simulink model "SF002A_Rtn"  (R2013b)
settings: Solver=FixedStepDiscrete  SolverMode=SingleTasking  StartTime=0.0  StopTime=1  FixedStep=0.002  RelTol=1e-3
values from neighbouring files (symbols this model uses):
  ARCHGLBPRM_2MILLISEC_SEC_F32 = DataDict.Constant    [SF002A_Rtn_DataDict.m]
  FLTINJ_RTN_RTNCMD = DataDict.Constant    [SF002A_Rtn_DataDict.m]
  RtnHwAuthySlew = DataDict.Calibration    [SF002A_Rtn_DataDict.m]
  RtnOffsRng = DataDict.Calibration    [SF002A_Rtn_DataDict.m]
  RtnOffsSlew = DataDict.Calibration    [SF002A_Rtn_DataDict.m]
libraries: FloatToFixd x8, FixdToFloat x5, NxtrLim x4, NxtrAbslt x3, BilnrIntrpnMplX x3, LnrIntrpn x2, simulink x1, NxtrSign x1
settings Model: Creator=tz5743  LastModifiedBy=XZB1DB
settings SolverCC: AutoInsertRateTranBlk=on  InsertRTBMode=Always
settings DataIOCC: LimitDataPoints=off  SaveFormat=Structure  ReturnWorkspaceOutputs=on
settings OptimizationCC: BlockReduction=off  InlineParams=on  ZeroExternalMemoryAtStartup=off  ZeroInternalMemoryAtStartup=off  OptimizeModelRefInitCode=on  LifeSpan=1
settings DebuggingCC: SignalInfNanChecking=error  SignalRangeChecking=warning  UnderspecifiedInitializationDetection=Simplified  SolverPrmCheckMsg=error  InheritedTsInSrcMsg=error  DiscreteInheritContinuousMsg=error  SingleTaskRateTransMsg=error  TasksWithSamePriorityMsg=error  SigSpecEnsureSampleTimeMsg=error  CheckMatrixSingularityMsg=error  ParameterUnderflowMsg=error  ParameterPrecisionLossMsg=error  ParameterTunabilityLossMsg=error  FixptConstUnderflowMsg=warning  FixptConstOverflowMsg=warning  VectorMatrixConversionMsg=error  SignalLabelMismatchMsg=error  UnconnectedInputMsg=error  UnconnectedOutputMsg=error  UnconnectedLineMsg=error  SFcnCompatibilityMsg=error  UniqueDataStoreMsg=warning  BusObjectLabelMismatch=error  RootOutportRequireBusObject=error  AssertControl=DisableAll  ModelReferenceIOMsg=error  ModelReferenceVersionMismatchMessage=warning  ModelReferenceIOMismatchMessage=error  ModelReferenceCSMismatchMessage=warning  ModelReferenceDataLoggingMessage=error  StateNameClashWarn=warning  StrictBusMsg=ErrorOnBusTreatedAsVector  NonBusSignalsTreatedAsBus=error  SFUnexpectedBacktrackingDiag=error  SFInvalidInputDataAccessInChartInitDiag=error  SFNoUnconditionalDefaultTransitionDiag=error  SFTransitionOutsideNaturalParentDiag=error  SFUnconditionalTransitionShadowingDiag=error  SFUndirectedBroadcastEventsDiag=error
settings ModelReferenceCC: ModelReferenceNumInstancesAllowed=Single
settings RTWCC: SystemTargetFile=autosar.tlc  GenCodeOnly=on  TemplateMakefile=ert_default_tmf  Description=AUTOSAR  GenerateReport=on  ProcessScript=autosar_make_rtw_hook  LaunchReport=on
settings CodeAppCC: GenerateComments=off  IgnoreCustomStorageClasses=off  CustomSymbolStrType=$N$R$M  CustomSymbolStrBlkIO=$N$M  SimulinkBlockComments=off
settings STFCustomTargetCC: ParMdlRefBuildCompliant=on  CompOptLevelCompliant=on  IncludeMdlTerminateFcn=off  CombineOutputUpdateFcns=on  SuppressErrorStatus=on  ERTFirstTimeCompliant=on  ERTCustomFileBanners=on  SupportNonFinite=off  SupportComplex=off  SupportContinuousTime=off  SupportNonInlinedSFcns=off  MATLABClassNameForMDSCustomization=Simulink.SoftwareTarget.ERTCustomization  AutosarCompliant=on  GRTInterface=off  SystemTargetFile=autosar.tlc
settings ERTTargetCC: CodeReplacementLibrary=ANSI_C  ConcurrentExecutionCompliant=off  IncludeMdlTerminateFcn=off  SuppressErrorStatus=on  SupportNonFinite=off  SupportComplex=off  ModelStepFunctionPrototypeControlCompliant=off  CPPClassGenCompliant=off  AutosarCompliant=on  InlinedParameterPlacement=NonHierarchical  ERTCustomFileTemplate=example_file_process.tlc  EnableUserReplacementTypes=on

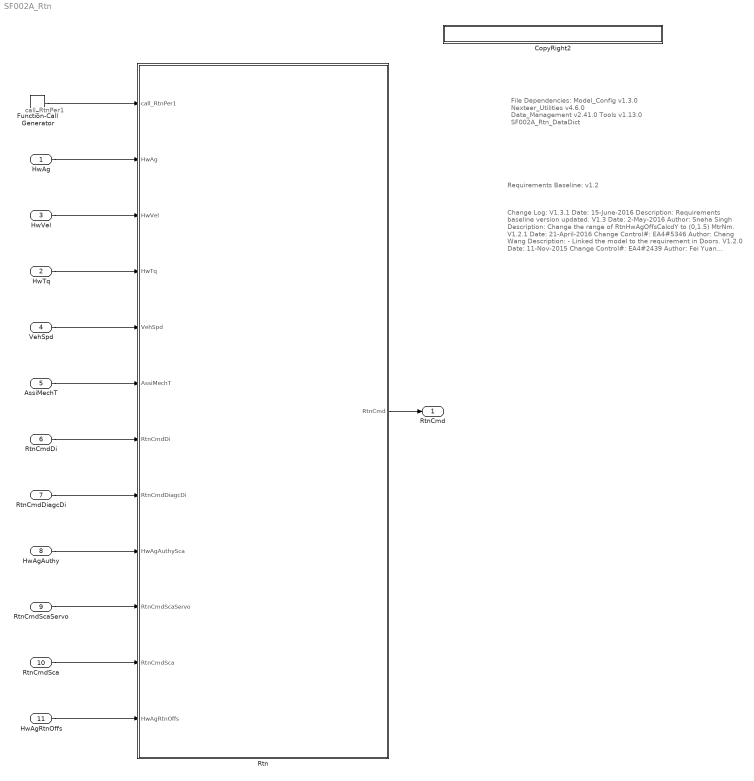
== system SF002A_Rtn ==
  note: call_RtnPer1
  note: File Dependencies:
      |
      | Model_Config v1.3.0
      | Nexteer_Utilities v4.6.0
      | Data_Management v2.41.0
      | Tools v1.13.0
      | SF002A_Rtn_DataDict
  note: Requirements Baseline: v1.2
  note: Change Log:
      |
      | V1.3.1
      | Date: 15-June-2016
      | Description:
      | Requirements baseline version updated.
      |
      | V1.3
      | Date: 2-May-2016
      | Author: Sneha Singh
      | Description:
      | Change the range of RtnHwAgOffsCalcdY to
      | (0,1.5) MtrNm.
      |
      | V1.2.1
      | Date: 21-April-2016
      | Change Control#: EA4#5346
      | Author: Chang Wang
      | Description:
      | - Linked the model to the requirement in Doors.
      |
      | V1.2.0
      | Date: 11-Nov-2015
      | Change Control#: EA4#2439
      | Author: Fei Yuan
      | Description:
      | Change the initial value of RtnCmdScaServo to 1
      |
      | V1.1.0
      | Date:29-Oct-2015
      | Change Control#: EA4#2248
      | Author : Sudeep Shankar
      | Description:
      | HwTq and HwVel changed to absolute values
      | before float to unsigned int conversion to fix
      | floating point error.
      |
      | v1.0.0
      | Date: 18-Jun-2015
      | Change Control #: EA4#759
      | DRW:  Sudeep Shankar
      | Description:
      | - Initial Release
  HwAg : Inport  RequirementInfo={'linktype_rmi_doors' '0000a524 (/E-STEER Core/SubSystem Specifications/Application Functions/SF002A Return)' '#SF002A_159' 'true' 'REQ:SF002A_159' '' } %GIDa_ca9d562d_6fa6_4620_b7e9_0be4ef6b3256
  HwTq : Inport  RequirementInfo={'linktype_rmi_doors' '0000a524 (/E-STEER Core/SubSystem Specifications/Application Functions/SF002A Return)' '#SF002A_161' 'true' 'REQ:SF002A_161' '' } %GIDa_270472cb_7f1b_499d_b316_9d3a4d63b4ae  Port=2
  HwVel : Inport  RequirementInfo={'linktype_rmi_doors' '0000a524 (/E-STEER Core/SubSystem Specifications/Application Functions/SF002A Return)' '#SF002A_160' 'true' 'REQ:SF002A_160' '' } %GIDa_baf48a56_f0cb_4bf9_a471_e23550366fc3  Port=3
  VehSpd : Inport  RequirementInfo={'linktype_rmi_doors' '0000a524 (/E-STEER Core/SubSystem Specifications/Application Functions/SF002A Return)' '#SF002A_162' 'true' 'REQ:SF002A_162' '' } %GIDa_bbc4534a_439c_4303_b734_20c92152eed5  Port=4
  AssiMechT : Inport  RequirementInfo={'linktype_rmi_doors' '0000a524 (/E-STEER Core/SubSystem Specifications/Application Functions/SF002A Return)' '#SF002A_163' 'true' 'REQ:SF002A_163' '' } %GIDa_7c5d29d7_e5a1_483a_8b5e_5f7fb39cc9db  Port=5
  RtnCmdDi : Inport  RequirementInfo={'linktype_rmi_doors' '0000a524 (/E-STEER Core/SubSystem Specifications/Application Functions/SF002A Return)' '#SF002A_164' 'true' 'REQ:SF002A_164' '' } %GIDa_de28c24d_f087_49cf_b2a4_d8c99114b430  Port=6
  RtnCmdDiagcDi : Inport  RequirementInfo={'linktype_rmi_doors' '0000a524 (/E-STEER Core/SubSystem Specifications/Application Functions/SF002A Return)' '#SF002A_165' 'true' 'REQ:SF002A_165' '' } %GIDa_ba846f76_0715_4d73_996c_66d22bdcf12b  Port=7
  HwAgAuthy : Inport  RequirementInfo={'linktype_rmi_doors' '0000a524 (/E-STEER Core/SubSystem Specifications/Application Functions/SF002A Return)' '#SF002A_166' 'true' 'REQ:SF002A_166' '' } %GIDa_5832e332_1aac_4b18_b389_bf82018842e7  Port=8
  RtnCmdScaServo : Inport  RequirementInfo={'linktype_rmi_doors' '0000a524 (/E-STEER Core/SubSystem Specifications/Application Functions/SF002A Return)' '#SF002A_167' 'true' 'REQ:SF002A_167' '' } %GIDa_ed132ec2_d50e_44ae_b5b8_67025ec0ffe6  Port=9
  RtnCmdSca : Inport  RequirementInfo={'linktype_rmi_doors' '0000a524 (/E-STEER Core/SubSystem Specifications/Application Functions/SF002A Return)' '#SF002A_168' 'true' 'REQ:SF002A_168' '' } %GIDa_5ecd380a_25d4_4e78_abc9_382ca1348921  Port=10
  HwAgRtnOffs : Inport  RequirementInfo={'linktype_rmi_doors' '0000a524 (/E-STEER Core/SubSystem Specifications/Application Functions/SF002A Return)' '#SF002A_169' 'true' 'REQ:SF002A_169' '' } %GIDa_4cf8cc8a_4d33_4739_b48e_beac64132d5a  Port=11
  CopyRight2 : Subsystem  Description=|  mask(Copyright Information){none=on}
      | Copyright info block.                                               
      |                                                                     
      | Place copyright information at the top of every subsystem in design.
      mask prompts: none "No parameters"
      mask help: Place copyright information at the top of every subsystem in design.
      mask Display:
      | NxtrConf = 'Nexteer Confidential';
      | 
      | sys = bdroot; %handle for the current model ("system")
      | first = get_param(sys,'Created');
      | if(isempty(first))
      |     first = datestr(now,'yyyy');
      | else
      |     first = first(end-3:end);  %year is last four digits
      | end
      | 
      | last = get_param(sys,'LastModifiedDate');
      | if isempty(last)
      |     last = datestr(now,'yyyy');
      | else
      |     last = last(end-3:end);
      | end
      | 
      | if strcmp(first,last)
      |     fprintf('%s -- Copyright %s Nexteer',NxtrConf,first)
      | else
      |     fprintf('%s -- %s%s- %s Nexteer',NxtrConf,char(169),first,last)
      | end
  Function-Call Generator : simulink/Ports & Subsystems/Function-Call Generator  RequirementInfo={} %GIDa_69592b82_c58d_4ec1_9fe3_c081b0261161  sample_time=0.002  numberOfIterations=1
  Rtn : Subsystem
  RtnCmd : Outport  RequirementInfo={'linktype_rmi_doors' '0000a524 (/E-STEER Core/SubSystem Specifications/Application Functions/SF002A Return)' '#SF002A_171' 'true' 'REQ:SF002A_171' '' } %GIDa_32987518_840e_4738_ba6a_c375293d3a7a
  wires:
  HwAg/1 -> Rtn/2(HwAg)
  HwVel/1 -> Rtn/3(HwVel)
  HwTq/1 -> Rtn/4(HwTq)
  VehSpd/1 -> Rtn/5(VehSpd)
  AssiMechT/1 -> Rtn/6(AssiMechT)
  RtnCmdDi/1 -> Rtn/7(RtnCmdDi)
  RtnCmdDiagcDi/1 -> Rtn/8(RtnCmdDiagcDi)
  HwAgAuthy/1 -> Rtn/9(HwAgAuthySca)
  RtnCmdScaServo/1 -> Rtn/10(RtnCmdScaServo)
  RtnCmdSca/1 -> Rtn/11(RtnCmdSca)
  HwAgRtnOffs/1 -> Rtn/12(HwAgRtnOffs)
  Rtn/1(RtnCmd) -> RtnCmd/1
  Function-Call Generator/1 -> Rtn/1(call_RtnPer1)

== system SF002A_Rtn/CopyRight2 ==

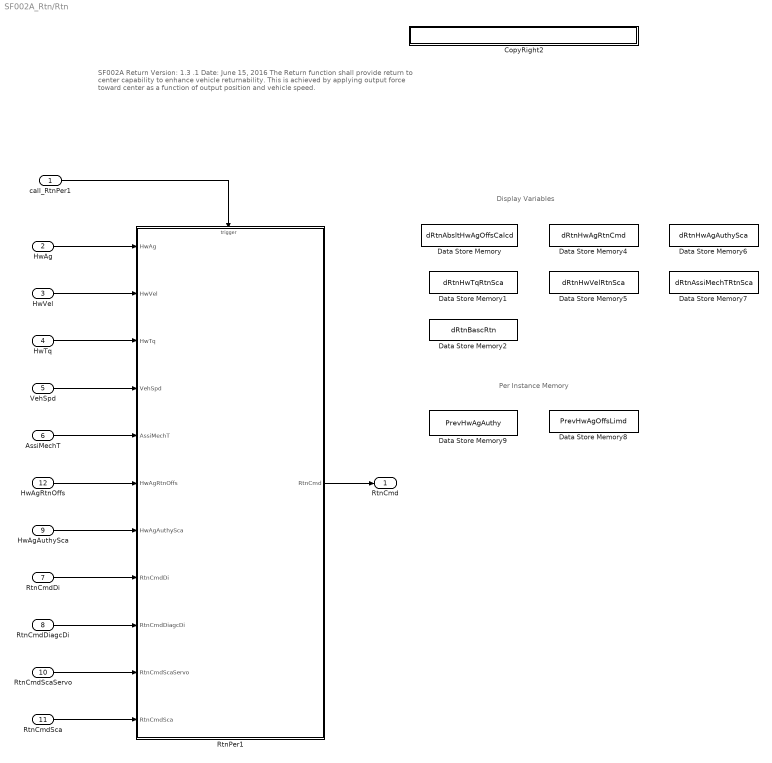
== system SF002A_Rtn/Rtn ==
  note: Per Instance Memory
  note: Display Variables
  note: SF002A Return       Version: 1.3 .1                                                    Date: June 15, 2016
      |
      | The Return function shall provide return to center capability to enhance vehicle returnability.
      | This is achieved by applying output force toward center as a function of output position and
      | vehicle speed.
  call_RtnPer1 : Inport
  HwAg : Inport  RequirementInfo={} %GIDa_81f6b954_2096_4808_9308_111896067df5  Port=2
  HwVel : Inport  RequirementInfo={} %GIDa_c3703c3f_c0e7_449a_8c9c_49994e2a0764  Port=3
  HwTq : Inport  RequirementInfo={} %GIDa_5aef1dee_ffa2_4027_a66e_3b3fd1650829  Port=4
  VehSpd : Inport  RequirementInfo={} %GIDa_5b3b3cf4_de38_4bc4_96c0_03a7b893fecb  Port=5
  AssiMechT : Inport  RequirementInfo={} %GIDa_63965e99_8cd9_4f5a_a8f1_ab380e00a545  Port=6
  RtnCmdDi : Inport  RequirementInfo={} %GIDa_5f11c497_b3cf_4940_a418_441be7e406df  Port=7
  RtnCmdDiagcDi : Inport  RequirementInfo={} %GIDa_42044fc9_5ea7_4c65_87aa_626e1dc46c63  Port=8
  HwAgAuthySca : Inport  RequirementInfo={} %GIDa_9af6312e_2c94_46c3_8264_c004198b3d25  Port=9
  RtnCmdScaServo : Inport  RequirementInfo={} %GIDa_cf95d922_a662_4add_b87b_c0abf245239e  Port=10
  RtnCmdSca : Inport  RequirementInfo={} %GIDa_d5119aae_365f_4c0e_b544_e70e493d88e1  Port=11
  HwAgRtnOffs : Inport  RequirementInfo={} %GIDa_3b2239f5_93a1_48f2_b8ad_42fbfe65ccd3  Port=12
  CopyRight2 : Subsystem  Description=|  mask(Copyright Information){none=on}
      | Copyright info block.                                               
      |                                                                     
      | Place copyright information at the top of every subsystem in design.
      mask prompts: none "No parameters"
      mask help: Place copyright information at the top of every subsystem in design.
      mask Display:
      | NxtrConf = 'Nexteer Confidential';
      | 
      | sys = bdroot; %handle for the current model ("system")
      | first = get_param(sys,'Created');
      | if(isempty(first))
      |     first = datestr(now,'yyyy');
      | else
      |     first = first(end-3:end);  %year is last four digits
      | end
      | 
      | last = get_param(sys,'LastModifiedDate');
      | if isempty(last)
      |     last = datestr(now,'yyyy');
      | else
      |     last = last(end-3:end);
      | end
      | 
      | if strcmp(first,last)
      |     fprintf('%s -- Copyright %s Nexteer',NxtrConf,first)
      | else
      |     fprintf('%s -- %s%s- %s Nexteer',NxtrConf,char(169),first,last)
      | end
  Data Store Memory : DataStoreMemory  DataStoreName=dRtnAbsltHwAgOffsCalcd  ReadBeforeWriteMsg=warning  WriteAfterWriteMsg=warning  WriteAfterReadMsg=warning  StateMustResolveToSignalObject=on
  Data Store Memory1 : DataStoreMemory  DataStoreName=dRtnHwTqRtnSca  ReadBeforeWriteMsg=warning  WriteAfterWriteMsg=warning  WriteAfterReadMsg=warning  StateMustResolveToSignalObject=on
  Data Store Memory2 : DataStoreMemory  DataStoreName=dRtnBascRtn  ReadBeforeWriteMsg=warning  WriteAfterWriteMsg=warning  WriteAfterReadMsg=warning  StateMustResolveToSignalObject=on
  Data Store Memory4 : DataStoreMemory  DataStoreName=dRtnHwAgRtnCmd  ReadBeforeWriteMsg=warning  WriteAfterWriteMsg=warning  WriteAfterReadMsg=warning  StateMustResolveToSignalObject=on
  Data Store Memory5 : DataStoreMemory  DataStoreName=dRtnHwVelRtnSca  ReadBeforeWriteMsg=warning  WriteAfterWriteMsg=warning  WriteAfterReadMsg=warning  StateMustResolveToSignalObject=on
  Data Store Memory6 : DataStoreMemory  DataStoreName=dRtnHwAgAuthySca  ReadBeforeWriteMsg=warning  WriteAfterWriteMsg=warning  WriteAfterReadMsg=warning  StateMustResolveToSignalObject=on
  Data Store Memory7 : DataStoreMemory  DataStoreName=dRtnAssiMechTRtnSca  ReadBeforeWriteMsg=warning  WriteAfterWriteMsg=warning  WriteAfterReadMsg=warning  StateMustResolveToSignalObject=on
  Data Store Memory8 : DataStoreMemory  DataStoreName=PrevHwAgOffsLimd  StateMustResolveToSignalObject=on
  Data Store Memory9 : DataStoreMemory  DataStoreName=PrevHwAgAuthy  StateMustResolveToSignalObject=on
  RtnPer1 : Subsystem  TreatAsAtomicUnit=on
  RtnCmd : Outport  RequirementInfo={} %GIDa_05e2840d_7433_4fe4_a387_0e6fe9f74771
  wires:
  AssiMechT/1 -> RtnPer1/5(AssiMechT)
  HwAgRtnOffs/1 -> RtnPer1/6(HwAgRtnOffs)
  RtnPer1/1(RtnCmd) -> RtnCmd/1
  HwAg/1 -> RtnPer1/1(HwAg)
  VehSpd/1 -> RtnPer1/4(VehSpd)
  HwTq/1 -> RtnPer1/3(HwTq)
  HwVel/1 -> RtnPer1/2(HwVel)
  call_RtnPer1/1 -> RtnPer1/Trigger
  HwAgAuthySca/1 -> RtnPer1/7(HwAgAuthySca)
  RtnCmdDi/1 -> RtnPer1/8(RtnCmdDi)
  RtnCmdDiagcDi/1 -> RtnPer1/9(RtnCmdDiagcDi)
  RtnCmdSca/1 -> RtnPer1/11(RtnCmdSca)
  RtnCmdScaServo/1 -> RtnPer1/10(RtnCmdScaServo)

== system SF002A_Rtn/Rtn/CopyRight2 ==

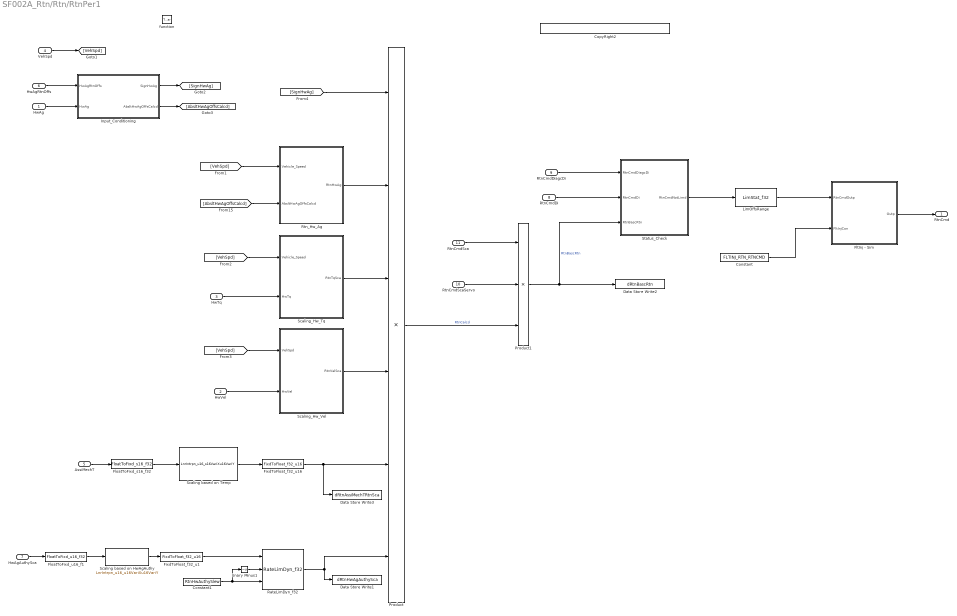
== system SF002A_Rtn/Rtn/RtnPer1 ==
  HwAg : Inport
  HwVel : Inport  Port=2
  HwTq : Inport  Port=3
  VehSpd : Inport  Port=4
  AssiMechT : Inport  Port=5
  HwAgRtnOffs : Inport  Port=6
  HwAgAuthySca : Inport  Port=7
  RtnCmdDi : Inport  Port=8
  RtnCmdDiagcDi : Inport  Port=9
  RtnCmdScaServo : Inport  Port=10
  RtnCmdSca : Inport  Port=11
  function : TriggerPort  TriggerType=function-call
  Constant : Constant  Value=FLTINJ_RTN_RTNCMD
  Constant1 : Constant  RequirementInfo={'linktype_rmi_doors' '0000a524 (/E-STEER Core/SubSystem Specifications/Application Functions/SF002A Return)' '#SF002A_206' 'true' 'REQ:SF002A_206' '' } %GIDa_f29b5096_6a10_4d8c_aa2b_ab6d9dbc01dd  Value=RtnHwAuthySlew
  CopyRight2 : Subsystem  Description=|  mask(Copyright Information){none=on}
      | Copyright info block.                                               
      |                                                                     
      | Place copyright information at the top of every subsystem in design.
      mask prompts: none "No parameters"
      mask help: Place copyright information at the top of every subsystem in design.
      mask Display:
      | NxtrConf = 'Nexteer Confidential';
      | 
      | sys = bdroot; %handle for the current model ("system")
      | first = get_param(sys,'Created');
      | if(isempty(first))
      |     first = datestr(now,'yyyy');
      | else
      |     first = first(end-3:end);  %year is last four digits
      | end
      | 
      | last = get_param(sys,'LastModifiedDate');
      | if isempty(last)
      |     last = datestr(now,'yyyy');
      | else
      |     last = last(end-3:end);
      | end
      | 
      | if strcmp(first,last)
      |     fprintf('%s -- Copyright %s Nexteer',NxtrConf,first)
      | else
      |     fprintf('%s -- %s%s- %s Nexteer',NxtrConf,char(169),first,last)
      | end
  Data Store Write1 : DataStoreWrite  DataStoreName=dRtnHwAgAuthySca
  Data Store Write2 : DataStoreWrite  DataStoreName=dRtnBascRtn
  Data Store Write3 : DataStoreWrite  DataStoreName=dRtnAssiMechTRtnSca
  FixdToFloat_f32_u1 : FixdToFloat/FixdToFloat_f32_u16  RequirementInfo={'linktype_rmi_doors' '0000a524 (/E-STEER Core/SubSystem Specifications/Application Functions/SF002A Return)' '#SF002A_205' 'true' 'REQ:SF002A_205' '' } %GIDa_b2f13837_bf2e_4759_92c8_f7ebb739a05c  Param1=7
  FixdToFloat_f32_u16 : FixdToFloat/FixdToFloat_f32_u16  RequirementInfo={'linktype_rmi_doors' '0000a524 (/E-STEER Core/SubSystem Specifications/Application Functions/SF002A Return)' '#SF002A_204' 'true' 'REQ:SF002A_204' '' } %GIDa_82025f1b_559c_4aab_bbbd_02cf94200a87  Param1=8
  FloatToFixd_s16_f32 : FloatToFixd/FloatToFixd_s16_f32  RequirementInfo={'linktype_rmi_doors' '0000a524 (/E-STEER Core/SubSystem Specifications/Application Functions/SF002A Return)' '#SF002A_204' 'true' 'REQ:SF002A_204' '' } %GIDa_56e826a7_394e_467a_81db_778c5b532e30  Param1=4
  FloatToFixd_u16_f1 : FloatToFixd/FloatToFixd_u16_f32  RequirementInfo={'linktype_rmi_doors' '0000a524 (/E-STEER Core/SubSystem Specifications/Application Functions/SF002A Return)' '#SF002A_205' 'true' 'REQ:SF002A_205' '' } %GIDa_026014ca_9083_4924_b7c0_5d559a60553d  Param1=8
  FltInj - Sim : Subsystem  TreatAsAtomicUnit=on  VariantControl=FltInj_sim  mask(Fault_Injection){}
      mask help: Fault Injection is a simulation only block for EA4 programs.
  Input_Conditioning : Subsystem  RequirementInfo={} %GIDa_067d012a_6457_4c55_9353_da0c0471b184
  LimOffsRange : NxtrLim/LimStat_f32  RequirementInfo={'linktype_rmi_doors' '0000a524 (/E-STEER Core/SubSystem Specifications/Application Functions/SF002A Return)' '#SF002A_212' 'true' 'REQ:SF002A_212' '' ; 'linktype_rmi_doors' '0000a524 (/E-STEER Core/SubSystem Specifications/Application Functions/SF002A Return)' '#SF002A_213' 'true' 'REQ:SF002A_213' '' } %GIDa_ab23da02_3b34_46cd_b196_7f8073eb848d  LoLim=SYSGLBPRM_MOTTQCMDLOLIM_MOTNWTMTR_F32  HiLim=SYSGLBPRM_MOTTQCMDHILIM_MOTNWTMTR_F32
      settings: AttributesFormatString=|
      | Low Limit: %<LoLim>
      | High Limit:%<HiLim>
  Product : Product  RequirementInfo={'linktype_rmi_doors' '0000a524 (/E-STEER Core/SubSystem Specifications/Application Functions/SF002A Return)' '#SF002A_207' 'true' 'REQ:SF002A_207' '' ; 'linktype_rmi_doors' '0000a524 (/E-STEER Core/SubSystem Specifications/Application Functions/SF002A Return)' '#SF002A_208' 'true' 'REQ:SF002A_208' '' } %GIDa_08f8f894_2fa8_4f72_bac9_f7575f211a8c  Inputs=6  RndMeth=Zero
  Product1 : Product  RequirementInfo={'linktype_rmi_doors' '0000a524 (/E-STEER Core/SubSystem Specifications/Application Functions/SF002A Return)' '#SF002A_207' 'true' 'REQ:SF002A_207' '' } %GIDa_71e52ba4_2843_42bc_8970_a10228086c20  Inputs=3  RndMeth=Zero
  RateLimDyn_f32 : NxtrLim/RateLimDyn_f32  RequirementInfo={'linktype_rmi_doors' '0000a524 (/E-STEER Core/SubSystem Specifications/Application Functions/SF002A Return)' '#SF002A_206' 'true' 'REQ:SF002A_206' '' } %GIDa_b7a544e9_f336_4c69_9d45_b0b4739fef51  StVar=PrevHwAgAuthy  Ts=ARCHGLBPRM_2MILLISEC_SEC_F32
      settings: AttributesFormatString=StVar: %<StVar>
  Rtn_Hw_Ag : Subsystem
  Scaling based on HwAgAuthy : LnrIntrpn/LnrIntrpn_u16_u16VariXu16VariY  RequirementInfo={'linktype_rmi_doors' '0000a524 (/E-STEER Core/SubSystem Specifications/Application Functions/SF002A Return)' '#SF002A_205' 'true' 'REQ:SF002A_205' '' } %GIDa_a2e059e5_fe33_4929_8913_41229897d28b  XTbl=RtnHwAuthyScaX  YTbl=RtnHwAuthyScaY
      settings: AttributesFormatString=Lnr ( u16VariX , u16VariY )
  Scaling based on Temp : LnrIntrpn/LnrIntrpn_u16_s16VariXu16VariY  RequirementInfo={'linktype_rmi_doors' '0000a524 (/E-STEER Core/SubSystem Specifications/Application Functions/SF002A Return)' '#SF002A_204' 'true' 'REQ:SF002A_204' '' } %GIDa_a7aa3a35_56d3_48d3_9473_6da7fb71fcbd  XTbl=RtnTScaX  YTbl=RtnTScaY
      settings: AttributesFormatString=Lnr ( s16VariX , u16VariY )
  Scaling_Hw_Tq : Subsystem
  Scaling_Hw_Vel : Subsystem
  Status_Check : Subsystem
  Unary Minus1 : UnaryMinus  RequirementInfo={'linktype_rmi_doors' '0000a524 (/E-STEER Core/SubSystem Specifications/Application Functions/SF002A Return)' '#SF002A_206' 'true' 'REQ:SF002A_206' '' } %GIDa_c50e97ce_443b_433d_b8c3_12b3522cf517
  RtnCmd : Outport
  wires:
  VehSpd/1 -> [VehSpd]
  HwAgRtnOffs/1 -> Input_Conditioning/1(HwAgRtnOffs)
  HwAg/1 -> Input_Conditioning/2(HwAg)
  Input_Conditioning/2(AbsltHwAgOffsCalcd) -> [AbsltHwAgOffsCalcd]
  Input_Conditioning/1(SignHwAg) -> [SignHwAg]
  [VehSpd] -> Rtn_Hw_Ag/1(Vehicle_Speed)
  [AbsltHwAgOffsCalcd] -> Rtn_Hw_Ag/2(AbsltHwAgOffsCalcd)
  [VehSpd] -> Scaling_Hw_Tq/1(Vehicle_Speed)
  HwTq/1 -> Scaling_Hw_Tq/2(HwTq)
  HwVel/1 -> Scaling_Hw_Vel/2(HwVel)
  [VehSpd] -> Scaling_Hw_Vel/1(VehSpd)
  [SignHwAg] -> Product/1
  Rtn_Hw_Ag/1(RtnHwAg) -> Product/2
  Scaling_Hw_Tq/1(RtnTqSca) -> Product/3
  Scaling_Hw_Vel/1(RtnVelSca) -> Product/4
  Scaling based on Temp/1 -> FixdToFloat_f32_u16/1
  RateLimDyn_f32/1 -> Product/6, Data Store Write1/1
  RtnCmdScaServo/1 -> Product1/2
  RtnCmdSca/1 -> Product1/1
  Product/1 -> Product1/3  "RtnCalcd"
  RtnCmdDiagcDi/1 -> Status_Check/1(RtnCmdDiagcDi)
  RtnCmdDi/1 -> Status_Check/2(RtnCmdDi)
  Product1/1 -> Data Store Write2/1, Status_Check/3(RtnBascRtn)  "RtnBascRtn"
  Status_Check/1(RtnCmdNotLimd) -> LimOffsRange/1
  AssiMechT/1 -> FloatToFixd_s16_f32/1
  FixdToFloat_f32_u16/1 -> Data Store Write3/1, Product/5
  FloatToFixd_s16_f32/1 -> Scaling based on Temp/1
  HwAgAuthySca/1 -> FloatToFixd_u16_f1/1
  FloatToFixd_u16_f1/1 -> Scaling based on HwAgAuthy/1
  Scaling based on HwAgAuthy/1 -> FixdToFloat_f32_u1/1
  FixdToFloat_f32_u1/1 -> RateLimDyn_f32/1
  Unary Minus1/1 -> RateLimDyn_f32/2
  Constant1/1 -> RateLimDyn_f32/3, Unary Minus1/1
  LimOffsRange/1 -> FltInj - Sim/1(RtnCmdOutp)
  FltInj - Sim/1(Outp) -> RtnCmd/1
  Constant/1 -> FltInj - Sim/2(FltInjCon)

== system SF002A_Rtn/Rtn/RtnPer1/CopyRight2 ==

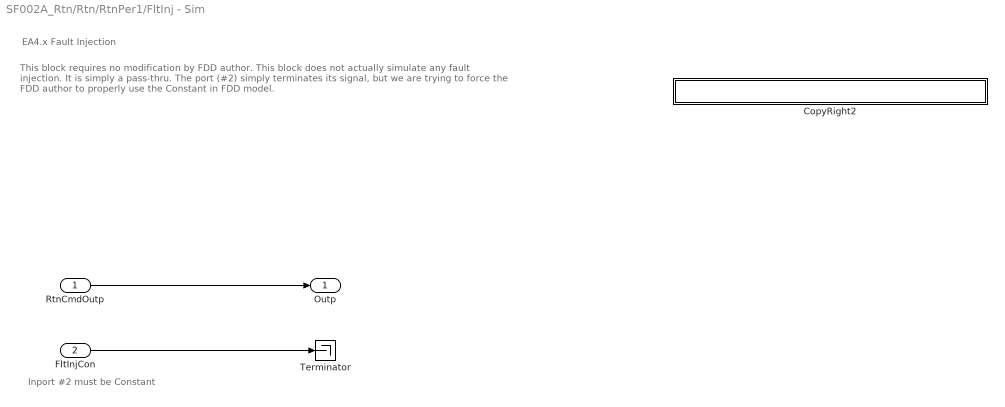
== system SF002A_Rtn/Rtn/RtnPer1/FltInj - Sim ==
  note: Inport #2 must be Constant
  note: EA4.x Fault Injection
  note: This block requires no modification by FDD author.
      |
      | This block does not actually simulate any fault injection.  It is simply a pass-thru.
      |
      | The port (#2) simply terminates its signal, but we are trying to force the FDD author
      | to properly use the Constant in FDD model.
  RtnCmdOutp : Inport
  FltInjCon : Inport  Port=2
  CopyRight2 : Subsystem  Description=|  mask(Copyright Information){none=on}
      | Copyright info block.                                               
      |                                                                     
      | Place copyright information at the top of every subsystem in design.
      mask prompts: none "No parameters"
      mask help: Place copyright information at the top of every subsystem in design.
      mask Display:
      | NxtrConf = 'Nexteer Confidential';
      | 
      | sys = bdroot; %handle for the current model ("system")
      | first = get_param(sys,'Created');
      | if(isempty(first))
      |     first = datestr(now,'yyyy');
      | else
      |     first = first(end-3:end);  %year is last four digits
      | end
      | 
      | last = get_param(sys,'LastModifiedDate');
      | if isempty(last)
      |     last = datestr(now,'yyyy');
      | else
      |     last = last(end-3:end);
      | end
      | 
      | if strcmp(first,last)
      |     fprintf('%s -- Copyright %s Nexteer',NxtrConf,first)
      | else
      |     fprintf('%s -- %s%s- %s Nexteer',NxtrConf,char(169),first,last)
      | end
  Terminator : Terminator
  Outp : Outport
  wires:
  FltInjCon/1 -> Terminator/1
  RtnCmdOutp/1 -> Outp/1

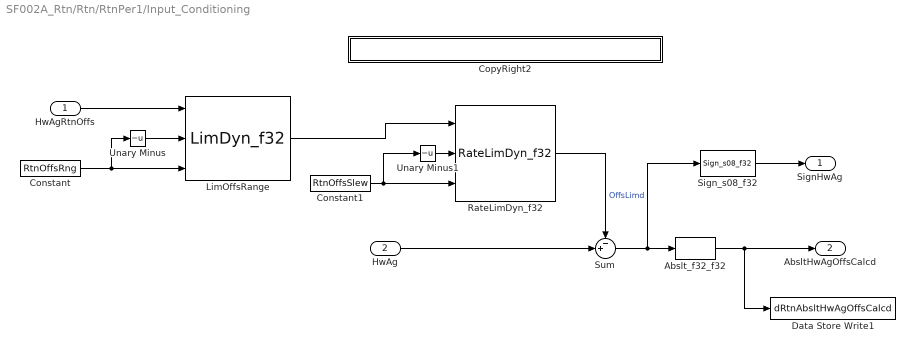
== system SF002A_Rtn/Rtn/RtnPer1/Input_Conditioning ==
  HwAgRtnOffs : Inport
  HwAg : Inport  Port=2
  Abslt_f32_f32 : NxtrAbslt/Abslt_f32_f32  RequirementInfo={'linktype_rmi_doors' '0000a524 (/E-STEER Core/SubSystem Specifications/Application Functions/SF002A Return)' '#SF002A_197' 'true' 'REQ:SF002A_197' '' } %GIDa_f9a85ec3_0f42_43d5_84e4_06570ad0613c  SFunctionSpec=single y1 = Abslt_f32_f32(single u1)
      settings: AttributesFormatString=%<Name>
  Constant : Constant  RequirementInfo={'linktype_rmi_doors' '0000a524 (/E-STEER Core/SubSystem Specifications/Application Functions/SF002A Return)' '#SF002A_194' 'true' 'REQ:SF002A_194' '' } %GIDa_47c6473a_a3a8_43c7_b9c8_d6bfcb974b57  Value=RtnOffsRng
  Constant1 : Constant  RequirementInfo={'linktype_rmi_doors' '0000a524 (/E-STEER Core/SubSystem Specifications/Application Functions/SF002A Return)' '#SF002A_195' 'true' 'REQ:SF002A_195' '' } %GIDa_e782450b_59be_4266_9724_56dfccf39984  Value=RtnOffsSlew
  CopyRight2 : Subsystem  Description=|  mask(Copyright Information){none=on}
      | Copyright info block.                                               
      |                                                                     
      | Place copyright information at the top of every subsystem in design.
      mask prompts: none "No parameters"
      mask help: Place copyright information at the top of every subsystem in design.
      mask Display:
      | NxtrConf = 'Nexteer Confidential';
      | 
      | sys = bdroot; %handle for the current model ("system")
      | first = get_param(sys,'Created');
      | if(isempty(first))
      |     first = datestr(now,'yyyy');
      | else
      |     first = first(end-3:end);  %year is last four digits
      | end
      | 
      | last = get_param(sys,'LastModifiedDate');
      | if isempty(last)
      |     last = datestr(now,'yyyy');
      | else
      |     last = last(end-3:end);
      | end
      | 
      | if strcmp(first,last)
      |     fprintf('%s -- Copyright %s Nexteer',NxtrConf,first)
      | else
      |     fprintf('%s -- %s%s- %s Nexteer',NxtrConf,char(169),first,last)
      | end
  Data Store Write1 : DataStoreWrite  DataStoreName=dRtnAbsltHwAgOffsCalcd
  LimOffsRange : NxtrLim/LimDyn_f32  RequirementInfo={'linktype_rmi_doors' '0000a524 (/E-STEER Core/SubSystem Specifications/Application Functions/SF002A Return)' '#SF002A_194' 'true' 'REQ:SF002A_194' '' } %GIDa_85bc1fd3_7e14_407a_bc7a_7924c3a08418
  RateLimDyn_f32 : NxtrLim/RateLimDyn_f32  RequirementInfo={'linktype_rmi_doors' '0000a524 (/E-STEER Core/SubSystem Specifications/Application Functions/SF002A Return)' '#SF002A_195' 'true' 'REQ:SF002A_195' '' } %GIDa_e60042c2_6ce2_4a60_a0b4_7c4b4394d0c9  StVar=PrevHwAgOffsLimd  Ts=ARCHGLBPRM_2MILLISEC_SEC_F32
      settings: AttributesFormatString=StVar: %<StVar>
  Sign_s08_f32 : NxtrSign/Sign_s08_f32  RequirementInfo={'linktype_rmi_doors' '0000a524 (/E-STEER Core/SubSystem Specifications/Application Functions/SF002A Return)' '#SF002A_208' 'true' 'REQ:SF002A_208' '' } %GIDa_10b1a9d9_a7df_4faf_a482_b22c82ff0ae7  SFunctionSpec=int8 y1 = Sign_s08_f32(single u1)
  Sum : Sum  RequirementInfo={'linktype_rmi_doors' '0000a524 (/E-STEER Core/SubSystem Specifications/Application Functions/SF002A Return)' '#SF002A_196' 'true' 'REQ:SF002A_196' '' } %GIDa_16c85849_0e99_4f36_a806_f0935ec46d22  Inputs=-+|
  Unary Minus : UnaryMinus  RequirementInfo={'linktype_rmi_doors' '0000a524 (/E-STEER Core/SubSystem Specifications/Application Functions/SF002A Return)' '#SF002A_194' 'true' 'REQ:SF002A_194' '' } %GIDa_a37619e5_1ce1_4f29_a669_52166bac9dfe
  Unary Minus1 : UnaryMinus  RequirementInfo={'linktype_rmi_doors' '0000a524 (/E-STEER Core/SubSystem Specifications/Application Functions/SF002A Return)' '#SF002A_195' 'true' 'REQ:SF002A_195' '' } %GIDa_aa6ee714_135e_4a10_8925_8941c20ed98f
  SignHwAg : Outport
  AbsltHwAgOffsCalcd : Outport  Port=2
  wires:
  RateLimDyn_f32/1 -> Sum/1  "OffsLimd"
  HwAg/1 -> Sum/2
  Sum/1 -> Sign_s08_f32/1, Abslt_f32_f32/1
  HwAgRtnOffs/1 -> LimOffsRange/1
  Sign_s08_f32/1 -> SignHwAg/1
  Abslt_f32_f32/1 -> Data Store Write1/1, AbsltHwAgOffsCalcd/1
  Constant/1 -> LimOffsRange/3, Unary Minus/1
  Unary Minus/1 -> LimOffsRange/2
  LimOffsRange/1 -> RateLimDyn_f32/1
  Constant1/1 -> RateLimDyn_f32/3, Unary Minus1/1
  Unary Minus1/1 -> RateLimDyn_f32/2

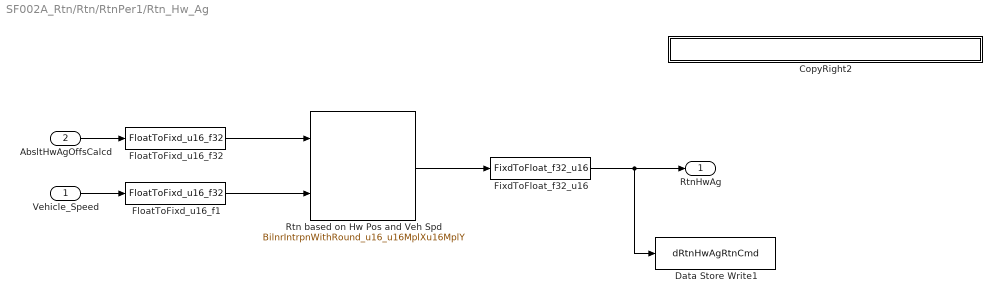
== system SF002A_Rtn/Rtn/RtnPer1/Rtn_Hw_Ag ==
  Vehicle_Speed : Inport
  AbsltHwAgOffsCalcd : Inport  Port=2
  CopyRight2 : Subsystem  Description=|  mask(Copyright Information){none=on}
      | Copyright info block.                                               
      |                                                                     
      | Place copyright information at the top of every subsystem in design.
      mask prompts: none "No parameters"
      mask help: Place copyright information at the top of every subsystem in design.
      mask Display:
      | NxtrConf = 'Nexteer Confidential';
      | 
      | sys = bdroot; %handle for the current model ("system")
      | first = get_param(sys,'Created');
      | if(isempty(first))
      |     first = datestr(now,'yyyy');
      | else
      |     first = first(end-3:end);  %year is last four digits
      | end
      | 
      | last = get_param(sys,'LastModifiedDate');
      | if isempty(last)
      |     last = datestr(now,'yyyy');
      | else
      |     last = last(end-3:end);
      | end
      | 
      | if strcmp(first,last)
      |     fprintf('%s -- Copyright %s Nexteer',NxtrConf,first)
      | else
      |     fprintf('%s -- %s%s- %s Nexteer',NxtrConf,char(169),first,last)
      | end
  Data Store Write1 : DataStoreWrite  DataStoreName=dRtnHwAgRtnCmd
  FixdToFloat_f32_u16 : FixdToFloat/FixdToFloat_f32_u16  RequirementInfo={'linktype_rmi_doors' '0000a524 (/E-STEER Core/SubSystem Specifications/Application Functions/SF002A Return)' '#SF002A_199' 'true' 'REQ:SF002A_199' '' } %GIDa_3cf2f3e4_d9fe_48dc_adbb_c76374402453  Param1=11
  FloatToFixd_u16_f1 : FloatToFixd/FloatToFixd_u16_f32  RequirementInfo={'linktype_rmi_doors' '0000a524 (/E-STEER Core/SubSystem Specifications/Application Functions/SF002A Return)' '#SF002A_199' 'true' 'REQ:SF002A_199' '' } %GIDa_61156389_bc0e_4aa8_8b6b_032d94995dae  Param1=7
  FloatToFixd_u16_f32 : FloatToFixd/FloatToFixd_u16_f32  RequirementInfo={'linktype_rmi_doors' '0000a524 (/E-STEER Core/SubSystem Specifications/Application Functions/SF002A Return)' '#SF002A_199' 'true' 'REQ:SF002A_199' '' } %GIDa_95321ca5_e4b7_4086_9e27_454ace152cf1  Param1=4
  Rtn based on Hw Pos and Veh Spd : BilnrIntrpnMplX/BilnrIntrpnWithRound_u16_u16MplXu16MplY  RequirementInfo={'linktype_rmi_doors' '0000a524 (/E-STEER Core/SubSystem Specifications/Application Functions/SF002A Return)' '#SF002A_199' 'true' 'REQ:SF002A_199' '' } %GIDa_9632ad9f_ee81_4170_a902_5fbb23a1dc2b  MplXTbl=RtnHwAgOffsCalcdX  MplYTbl=RtnHwAgOffsCalcdY  BilnrSelnTbl=RtnVehSpdSeln
      settings: AttributesFormatString=Bilnr ( u16MplX , u16MplY )
  RtnHwAg : Outport
  wires:
  Vehicle_Speed/1 -> FloatToFixd_u16_f1/1
  FloatToFixd_u16_f32/1 -> Rtn based on Hw Pos and Veh Spd/1
  AbsltHwAgOffsCalcd/1 -> FloatToFixd_u16_f32/1
  FixdToFloat_f32_u16/1 -> Data Store Write1/1, RtnHwAg/1
  FloatToFixd_u16_f1/1 -> Rtn based on Hw Pos and Veh Spd/2
  Rtn based on Hw Pos and Veh Spd/1 -> FixdToFloat_f32_u16/1

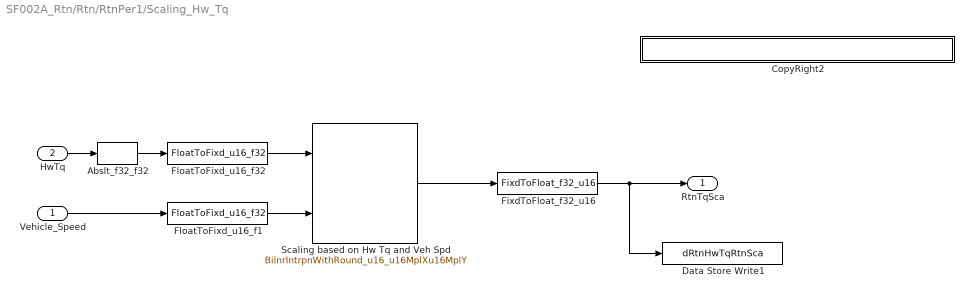
== system SF002A_Rtn/Rtn/RtnPer1/Scaling_Hw_Tq ==
  Vehicle_Speed : Inport
  HwTq : Inport  Port=2
  Abslt_f32_f32 : NxtrAbslt/Abslt_f32_f32  RequirementInfo={'linktype_rmi_doors' '0000a524 (/E-STEER Core/SubSystem Specifications/Application Functions/SF002A Return)' '#SF002A_202' 'true' 'REQ:SF002A_202' '' } %GIDa_d6e863f0_752f_43b9_aab3_d5f4a6f0f176  SFunctionSpec=single y1 = Abslt_f32_f32(single u1)
      settings: AttributesFormatString=%<Name>
  CopyRight2 : Subsystem  Description=|  mask(Copyright Information){none=on}
      | Copyright info block.                                               
      |                                                                     
      | Place copyright information at the top of every subsystem in design.
      mask prompts: none "No parameters"
      mask help: Place copyright information at the top of every subsystem in design.
      mask Display:
      | NxtrConf = 'Nexteer Confidential';
      | 
      | sys = bdroot; %handle for the current model ("system")
      | first = get_param(sys,'Created');
      | if(isempty(first))
      |     first = datestr(now,'yyyy');
      | else
      |     first = first(end-3:end);  %year is last four digits
      | end
      | 
      | last = get_param(sys,'LastModifiedDate');
      | if isempty(last)
      |     last = datestr(now,'yyyy');
      | else
      |     last = last(end-3:end);
      | end
      | 
      | if strcmp(first,last)
      |     fprintf('%s -- Copyright %s Nexteer',NxtrConf,first)
      | else
      |     fprintf('%s -- %s%s- %s Nexteer',NxtrConf,char(169),first,last)
      | end
  Data Store Write1 : DataStoreWrite  DataStoreName=dRtnHwTqRtnSca
  FixdToFloat_f32_u16 : FixdToFloat/FixdToFloat_f32_u16  RequirementInfo={'linktype_rmi_doors' '0000a524 (/E-STEER Core/SubSystem Specifications/Application Functions/SF002A Return)' '#SF002A_202' 'true' 'REQ:SF002A_202' '' } %GIDa_4082178c_4f0e_46bb_82f9_2524c4802890  Param1=8
  FloatToFixd_u16_f1 : FloatToFixd/FloatToFixd_u16_f32  RequirementInfo={'linktype_rmi_doors' '0000a524 (/E-STEER Core/SubSystem Specifications/Application Functions/SF002A Return)' '#SF002A_202' 'true' 'REQ:SF002A_202' '' } %GIDa_887a2362_f150_4659_9cfa_fa7edcfc4edd  Param1=7
  FloatToFixd_u16_f32 : FloatToFixd/FloatToFixd_u16_f32  RequirementInfo={'linktype_rmi_doors' '0000a524 (/E-STEER Core/SubSystem Specifications/Application Functions/SF002A Return)' '#SF002A_202' 'true' 'REQ:SF002A_202' '' } %GIDa_1a5e301e_d148_4ca7_a61b_6be7b1b61b63  Param1=8
  Scaling based on Hw Tq and Veh Spd : BilnrIntrpnMplX/BilnrIntrpnWithRound_u16_u16MplXu16MplY  RequirementInfo={'linktype_rmi_doors' '0000a524 (/E-STEER Core/SubSystem Specifications/Application Functions/SF002A Return)' '#SF002A_202' 'true' 'REQ:SF002A_202' '' } %GIDa_dd9cec9d_554f_4b6a_8068_650c9d9491fb  MplXTbl=RtnScaTqX  MplYTbl=RtnScaTqY  BilnrSelnTbl=RtnVehSpdSeln
      settings: AttributesFormatString=Bilnr ( u16MplX , u16MplY )
  RtnTqSca : Outport
  wires:
  FixdToFloat_f32_u16/1 -> Data Store Write1/1, RtnTqSca/1
  HwTq/1 -> Abslt_f32_f32/1
  FloatToFixd_u16_f32/1 -> Scaling based on Hw Tq and Veh Spd/1
  Vehicle_Speed/1 -> FloatToFixd_u16_f1/1
  FloatToFixd_u16_f1/1 -> Scaling based on Hw Tq and Veh Spd/2
  Scaling based on Hw Tq and Veh Spd/1 -> FixdToFloat_f32_u16/1
  Abslt_f32_f32/1 -> FloatToFixd_u16_f32/1

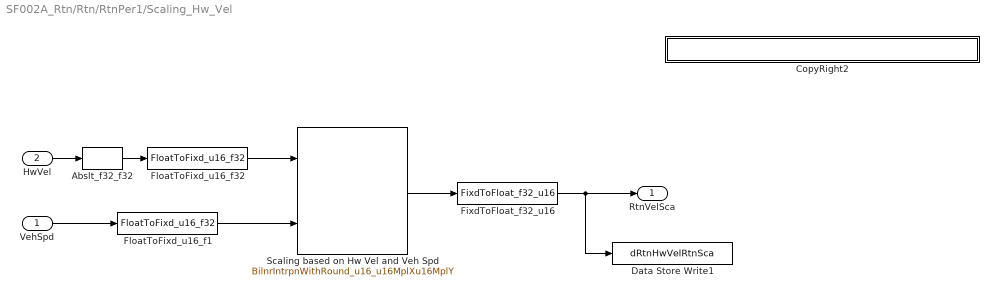
== system SF002A_Rtn/Rtn/RtnPer1/Scaling_Hw_Vel ==
  VehSpd : Inport
  HwVel : Inport  Port=2
  Abslt_f32_f32 : NxtrAbslt/Abslt_f32_f32  RequirementInfo={'linktype_rmi_doors' '0000a524 (/E-STEER Core/SubSystem Specifications/Application Functions/SF002A Return)' '#SF002A_203' 'true' 'REQ:SF002A_203' '' } %GIDa_4f140a35_909f_4123_902c_ff10627853cb  SFunctionSpec=single y1 = Abslt_f32_f32(single u1)
      settings: AttributesFormatString=%<Name>
  CopyRight2 : Subsystem  Description=|  mask(Copyright Information){none=on}
      | Copyright info block.                                               
      |                                                                     
      | Place copyright information at the top of every subsystem in design.
      mask prompts: none "No parameters"
      mask help: Place copyright information at the top of every subsystem in design.
      mask Display:
      | NxtrConf = 'Nexteer Confidential';
      | 
      | sys = bdroot; %handle for the current model ("system")
      | first = get_param(sys,'Created');
      | if(isempty(first))
      |     first = datestr(now,'yyyy');
      | else
      |     first = first(end-3:end);  %year is last four digits
      | end
      | 
      | last = get_param(sys,'LastModifiedDate');
      | if isempty(last)
      |     last = datestr(now,'yyyy');
      | else
      |     last = last(end-3:end);
      | end
      | 
      | if strcmp(first,last)
      |     fprintf('%s -- Copyright %s Nexteer',NxtrConf,first)
      | else
      |     fprintf('%s -- %s%s- %s Nexteer',NxtrConf,char(169),first,last)
      | end
  Data Store Write1 : DataStoreWrite  DataStoreName=dRtnHwVelRtnSca
  FixdToFloat_f32_u16 : FixdToFloat/FixdToFloat_f32_u16  RequirementInfo={'linktype_rmi_doors' '0000a524 (/E-STEER Core/SubSystem Specifications/Application Functions/SF002A Return)' '#SF002A_203' 'true' 'REQ:SF002A_203' '' } %GIDa_feae0ca5_21a8_44c5_90a5_83f5017ff4eb  Param1=8
  FloatToFixd_u16_f1 : FloatToFixd/FloatToFixd_u16_f32  RequirementInfo={'linktype_rmi_doors' '0000a524 (/E-STEER Core/SubSystem Specifications/Application Functions/SF002A Return)' '#SF002A_203' 'true' 'REQ:SF002A_203' '' } %GIDa_33dbaaae_2f0a_4d0b_a1d2_8019a1b100c9  Param1=7
  FloatToFixd_u16_f32 : FloatToFixd/FloatToFixd_u16_f32  RequirementInfo={'linktype_rmi_doors' '0000a524 (/E-STEER Core/SubSystem Specifications/Application Functions/SF002A Return)' '#SF002A_203' 'true' 'REQ:SF002A_203' '' } %GIDa_e3c79329_2c87_4229_b7b0_d6d44148f3d1  Param1=9
  Scaling based on Hw Vel and Veh Spd : BilnrIntrpnMplX/BilnrIntrpnWithRound_u16_u16MplXu16MplY  RequirementInfo={'linktype_rmi_doors' '0000a524 (/E-STEER Core/SubSystem Specifications/Application Functions/SF002A Return)' '#SF002A_203' 'true' 'REQ:SF002A_203' '' } %GIDa_69d8dc7d_44a4_47c3_9b35_8f8dbe547061  MplXTbl=RtnScaVelX  MplYTbl=RtnScaVelY  BilnrSelnTbl=RtnVehSpdSeln
      settings: AttributesFormatString=Bilnr ( u16MplX , u16MplY )
  RtnVelSca : Outport
  wires:
  VehSpd/1 -> FloatToFixd_u16_f1/1
  HwVel/1 -> Abslt_f32_f32/1
  FixdToFloat_f32_u16/1 -> Data Store Write1/1, RtnVelSca/1
  FloatToFixd_u16_f1/1 -> Scaling based on Hw Vel and Veh Spd/2
  FloatToFixd_u16_f32/1 -> Scaling based on Hw Vel and Veh Spd/1
  Scaling based on Hw Vel and Veh Spd/1 -> FixdToFloat_f32_u16/1
  Abslt_f32_f32/1 -> FloatToFixd_u16_f32/1

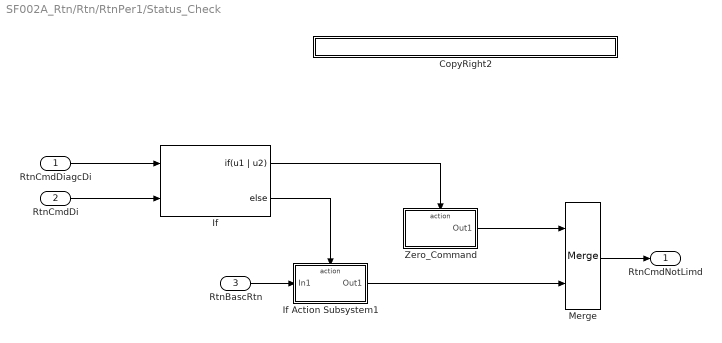
== system SF002A_Rtn/Rtn/RtnPer1/Status_Check ==
  RtnCmdDiagcDi : Inport
  RtnCmdDi : Inport  Port=2
  RtnBascRtn : Inport  Port=3
  CopyRight2 : Subsystem  Description=|  mask(Copyright Information){none=on}
      | Copyright info block.                                               
      |                                                                     
      | Place copyright information at the top of every subsystem in design.
      mask prompts: none "No parameters"
      mask help: Place copyright information at the top of every subsystem in design.
      mask Display:
      | NxtrConf = 'Nexteer Confidential';
      | 
      | sys = bdroot; %handle for the current model ("system")
      | first = get_param(sys,'Created');
      | if(isempty(first))
      |     first = datestr(now,'yyyy');
      | else
      |     first = first(end-3:end);  %year is last four digits
      | end
      | 
      | last = get_param(sys,'LastModifiedDate');
      | if isempty(last)
      |     last = datestr(now,'yyyy');
      | else
      |     last = last(end-3:end);
      | end
      | 
      | if strcmp(first,last)
      |     fprintf('%s -- Copyright %s Nexteer',NxtrConf,first)
      | else
      |     fprintf('%s -- %s%s- %s Nexteer',NxtrConf,char(169),first,last)
      | end
  If : If  RequirementInfo={'linktype_rmi_doors' '0000a524 (/E-STEER Core/SubSystem Specifications/Application Functions/SF002A Return)' '#SF002A_210' 'true' 'REQ:SF002A_210' '' ; 'linktype_rmi_doors' '0000a524 (/E-STEER Core/SubSystem Specifications/Application Functions/SF002A Return)' '#SF002A_229' 'true' 'REQ:SF002A_229' '' } %GIDa_b70a6fae_cb8b_4483_b7e7_25240ceafecb  NumInputs=2  IfExpression=u1 | u2
  If Action Subsystem1 : Subsystem  RequirementInfo={'linktype_rmi_doors' '0000a524 (/E-STEER Core/SubSystem Specifications/Application Functions/SF002A Return)' '#SF002A_229' 'true' 'REQ:SF002A_229' '' } %GIDa_0f5b89ad_9754_406d_bae3_388fd69f7b19  TreatAsAtomicUnit=on
  Merge : Merge  RequirementInfo={'linktype_rmi_doors' '0000a524 (/E-STEER Core/SubSystem Specifications/Application Functions/SF002A Return)' '#SF002A_210' 'true' 'REQ:SF002A_210' '' ; 'linktype_rmi_doors' '0000a524 (/E-STEER Core/SubSystem Specifications/Application Functions/SF002A Return)' '#SF002A_229' 'true' 'REQ:SF002A_229' '' } %GIDa_4bcad8da_a158_4a18_ab5d_11aaaf30a2a7
  Zero_Command : Subsystem  RequirementInfo={'linktype_rmi_doors' '0000a524 (/E-STEER Core/SubSystem Specifications/Application Functions/SF002A Return)' '#SF002A_210' 'true' 'REQ:SF002A_210' '' } %GIDa_595159e9_14e4_4547_a867_58be9411f91e  TreatAsAtomicUnit=on
  RtnCmdNotLimd : Outport
  wires:
  If/2 -> If Action Subsystem1/Action
  If/1 -> Zero_Command/Action
  RtnBascRtn/1 -> If Action Subsystem1/1(In1)
  If Action Subsystem1/1(Out1) -> Merge/2
  Zero_Command/1(Out1) -> Merge/1
  Merge/1 -> RtnCmdNotLimd/1
  RtnCmdDiagcDi/1 -> If/1
  RtnCmdDi/1 -> If/2

== system SF002A_Rtn/Rtn/RtnPer1/FltInj - Sim/CopyRight2 ==

== system SF002A_Rtn/Rtn/RtnPer1/Input_Conditioning/CopyRight2 ==

== system SF002A_Rtn/Rtn/RtnPer1/Rtn_Hw_Ag/CopyRight2 ==

== system SF002A_Rtn/Rtn/RtnPer1/Scaling_Hw_Tq/CopyRight2 ==

== system SF002A_Rtn/Rtn/RtnPer1/Scaling_Hw_Vel/CopyRight2 ==

== system SF002A_Rtn/Rtn/RtnPer1/Status_Check/CopyRight2 ==

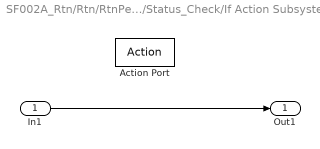
== system SF002A_Rtn/Rtn/RtnPer1/Status_Check/If Action Subsystem1 ==
  In1 : Inport
  Action Port : ActionPort  ActionType=else
  Out1 : Outport
  wires:
  In1/1 -> Out1/1

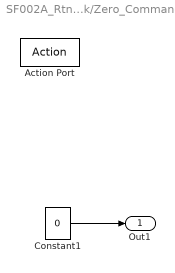
== system SF002A_Rtn/Rtn/RtnPer1/Status_Check/Zero_Command ==
  Action Port : ActionPort  ActionType=then
  Constant1 : Constant  RequirementInfo={} %GIDa_6ba828f0_41f8_4550_b05b_5bcdf21c98e7  Value=0  OutDataTypeStr=single
  Out1 : Outport
  wires:
  Constant1/1 -> Out1/1
